simulink model "Question_3"  (R2024b)
settings: Solver=VariableStepAuto  StartTime=0.0  StopTime=10.0  RelTol=1e-3
undefined symbols (not defined in the file): b1, b2, k, M1, M2
libraries: slpidlib x1
settings Model: Creator=Sagar  LastModifiedBy=Sagar

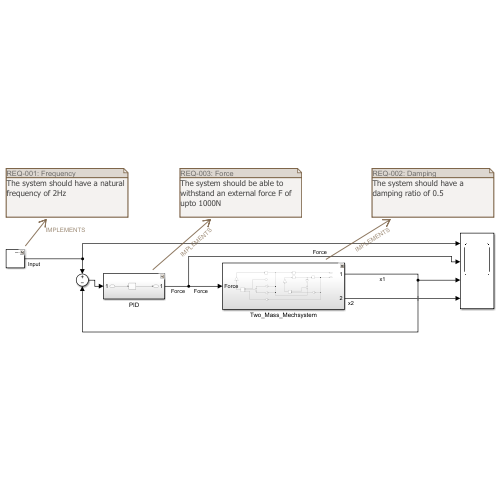
[thumbnail: Simulink's stored preview of the top-level diagram]
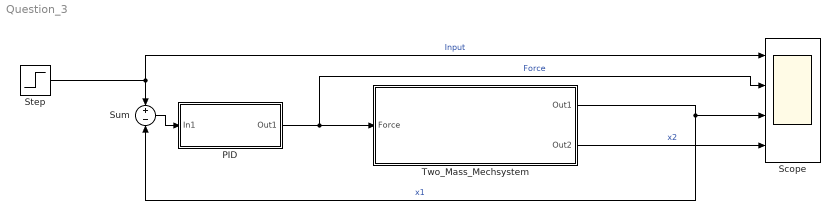
== system Question_3 ==
  PID : Subsystem
  Scope : Scope  NumInputPorts=4
  Step : Step  Time=2  After=3  SampleTime=0
  Sum : Sum  Inputs=+-
  Two_Mass_Mechsystem : Subsystem
  wires:
  Two_Mass_Mechsystem/2(Out2) -> Scope/4  "x2"
  PID/1(Out1) -> Scope/2, Two_Mass_Mechsystem/1(Force)  "Force"
  Sum/1 -> PID/1(In1)
  Two_Mass_Mechsystem/1(Out1) -> Sum/2, Scope/3  "x1"
  Step/1 -> Scope/1, Sum/1  "Input"

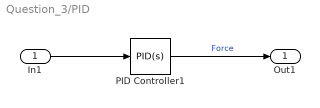
== system Question_3/PID ==
  In1 : Inport
  PID Controller1 : slpidlib/PID Controller  Controller=PID  Form=Parallel  TimeDomain=Continuous-time  UseExternalTs=off  SampleTime=-1  IntegratorMethod=Forward Euler  FilterMethod=Forward Euler  ControllerParametersSource=internal  P=314.829140399527  I=451.747100603338  UseKiTs=off  D=21.2834220388125  UseExternalDerivativeSource=off  N=1491.4635645043  UseFilter=on  TunerSelectOption=Transfer Function Based (PID Tuner App)  InitialConditionSource=internal  InitialConditionForIntegrator=0  InitialConditionForFilter=0  DifferentiatorICPrevScaledInput=0  ExternalReset=none  TrackingMode=off  Kt=1  LimitOutput=off  SatLimitsSource=internal  UpperSaturationLimit=inf  LowerSaturationLimit=-inf  LinearizeAsGain=on  AntiWindupMode=none  Kb=1  LimitIntegrator=off  UpperIntegratorSaturationLimit=inf  LowerIntegratorSaturationLimit=-inf  POutMin=[]  POutMax=[]  IOutMin=[]  IOutMax=[]  DOutMin=[]  DOutMax=[]  NOutMin=[]  NOutMax=[]  SumOutMin=[]  SumOutMax=[]  SaturationOutMin=[]  SaturationOutMax=[]  PParamMin=[]  PParamMax=[]  IParamMin=[]  IParamMax=[]  DParamMin=[]  DParamMax=[]  NParamMin=[]  NParamMax=[]  KbParamMin=[]  KbParamMax=[]  KtParamMin=[]  KtParamMax=[]  KbOutMin=[]  KbOutMax=[]  KtOutMin=[]  KtOutMax=[]  IntegratorOutMin=[]  IntegratorOutMax=[]  FilterOutMin=[]  FilterOutMax=[]  SumI1OutMin=[]  SumI1OutMax=[]  SumI2OutMin=[]  SumI2OutMax=[]  SumI3OutMin=[]  SumI3OutMax=[]  SumI4OutMin=[]  SumI4OutMax=[]  SumDOutMin=[]  SumDOutMax=[]  DifferentiatorOutMin=[]  DifferentiatorOutMax=[]  FilterDiffOutCoefMin=[]  FilterDiffOutCoefMax=[]  ReciprocalOutMin=[]  ReciprocalOutMax=[]  SumDenOutMin=[]  SumDenOutMax=[]  SumNumOutMin=[]  SumNumOutMax=[]  DivideOutMin=[]  DivideOutMax=[]  UdiffTsProdOutMin=[]  UdiffTsProdOutMax=[]  NTsProdOutMin=[]  NTsProdOutMax=[]  UintegralTsProdOutMin=[]  UintegralTsProdOutMax=[]  UngainTsProdOutMin=[]  UngainTsProdOutMax=[]  ClampingZeroOutDataTypeStr=Inherit: Inherit via back propagation  ClampingZeroOutMin=[]  ClampingZeroOutMax=[]  FilterDenConstantOutDataTypeStr=Inherit: Inherit via back propagation  FilterDenConstantOutMin=[]  FilterDenConstantOutMax=[]  PCopyOutDataTypeStr=Inherit: Inherit via back propagation  PCopyOutMin=[]  PCopyOutMax=[]  NCopyOutDataTypeStr=Inherit: Inherit via back propagation  NCopyOutMin=[]  NCopyOutMax=[]  IntegratorContinuousStateAttributes=''  IntegratorStateMustResolveToSignalObject=off  IntegratorRTWStateStorageClass=Auto  FilterContinuousStateAttributes=''  FilterStateMustResolveToSignalObject=off  FilterRTWStateStorageClass=Auto  ParallelPVariant=InternalParameters  IdealPVariant=Disabled  IVariant=InternalParameters  DVariant=InternalParameters  IntegratorVariant=Continuous  SatVariant=Disabled  AWVariant=Passthrough  PCopyVariant=Disabled  TRVariant=Disabled  FdbkBlocksVariant=Forward  IdealPFdbkVariant=Disabled  SatFdbkVariant=Disabled  DerivativeFilterVariant=ContFilter  NVariant=InternalParameters  NCopyVariant=Disabled  FilterICVariant=InternalICsFilter  IntegratorICVariant=InternalICs  ExternalResetVariant=Disabled  TRSumVariant=Passthrough  SumFdbkVariant=Disabled  SumVariant=Sum_PID  TsampFilterVariant=InternalTs  TsampNgainVariant=Passthrough  TsampIntegralVariant=Disabled_SignalSpec  ExternalSaturationOutDataTypeStr=Inherit: Same as second input  DerivativeSourceVariant=ErrorSignal  PreIntVariant=InternalPreInt
  Out1 : Outport
  wires:
  In1/1 -> PID Controller1/1
  PID Controller1/1 -> Out1/1  "Force"

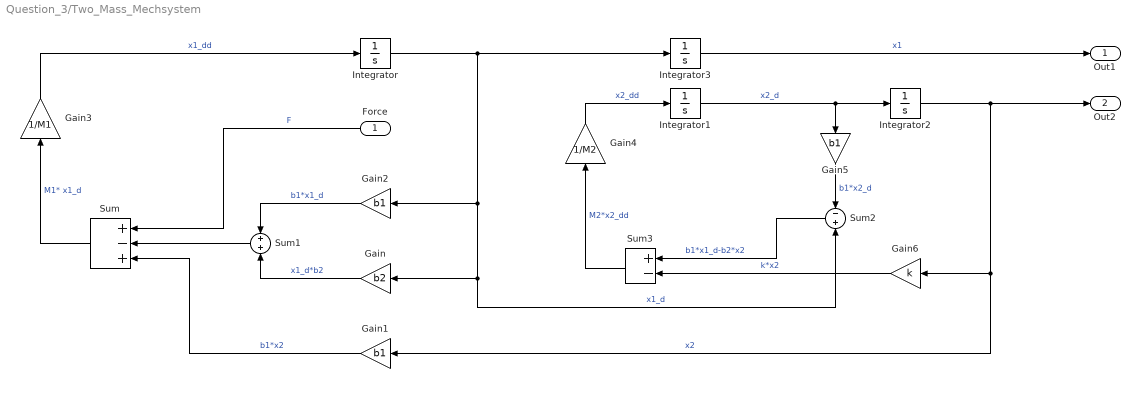
== system Question_3/Two_Mass_Mechsystem ==
  Force : Inport
  Gain : Gain  Gain=b2
  Gain1 : Gain  Gain=b1
  Gain2 : Gain  Gain=b1
  Gain3 : Gain  Gain=1/M1
  Gain4 : Gain  Gain=1/M2
  Gain5 : Gain  Gain=b1
  Gain6 : Gain  Gain=k
  Integrator{,1..3} (4 alike) : Integrator
  Sum : Sum  Inputs=+-+
  Sum1 : Sum
  Sum2 : Sum  Inputs=-+
  Sum3 : Sum  Inputs=+-
  Out1 : Outport
  Out2 : Outport  Port=2
  wires:
  Gain5/1 -> Sum2/1  "b1*x2_d"
  Gain1/1 -> Sum/3  "b1*x2"
  Sum3/1 -> Gain4/1  "M2*x2_dd"
  Sum2/1 -> Sum3/1  "b1*x1_d-b2*x2"
  Gain/1 -> Sum1/2  "x1_d*b2"
  Integrator/1 -> Integrator3/1, Gain2/1, Sum2/2, Gain/1  "x1_d"
  Integrator1/1 -> Integrator2/1, Gain5/1  "x2_d"
  Sum/1 -> Gain3/1  "M1* x1_d"
  Gain6/1 -> Sum3/2  "k*x2"
  Gain3/1 -> Integrator/1  "x1_dd"
  Integrator3/1 -> Out1/1  "x1"
  Gain2/1 -> Sum1/1  "b1*x1_d"
  Force/1 -> Sum/1  "F"
  Integrator2/1 -> Out2/1, Gain6/1, Gain1/1  "x2"
  Sum1/1 -> Sum/2
  Gain4/1 -> Integrator1/1  "x2_dd"
